simulink model "pulse_heating_official_spine_v04_git_recovery"  (R2025b)
settings: Solver=VariableStepAuto  StartTime=0.0  StopTime=0.001  RelTol=1e-3
PreLoadFcn:
  | addpath('C:\Users\ADMIN\Documents\MATLAB\Examples\R2025b\simscapeelectrical\BatteryThermalManagementExample');
  | addpath('C:\Users\ADMIN\Documents\MATLAB\Examples\R2025b\mcb\SIUnitsExample');
  | addpath('C:\Users\ADMIN\Documents\MATLAB\Examples\R2025b\simscapeelectrical\PMSMDriveThermalExample');
  | load_system('PMSMDriveThermal');
  | set_param('PMSMDriveThermal','SimscapeLogType','none','SimscapeLogSimulationStatistics','off');
  | set_param('PMSMDriveThermal','Dirty','off');
InitFcn:
  | addpath('C:\Users\ADMIN\Documents\MATLAB\Examples\R2025b\simscapeelectrical\BatteryThermalManagementExample');
  | addpath('C:\Users\ADMIN\Documents\MATLAB\Examples\R2025b\mcb\SIUnitsExample');
  | addpath('C:\Users\ADMIN\Documents\MATLAB\Examples\R2025b\simscapeelectrical\PMSMDriveThermalExample');
  | load_system('PMSMDriveThermal');
  | PMSMDriveThermalData;
  | mcb_pmsm_foc_qep_f28379d_SIUnit_data;
  | bw_i = (PI_params.Kp_i + pmsm.Rs) / pmsm.Ld;
  | pmsm.Rs = Rs; pmsm.Ld = Ld; pmsm.Lq = Lq; pmsm.p = N; pmsm.FluxPM = PM;
  | pmsm.J = J; pmsm.Ke = PM*N; pmsm.Kt = 1.5*N*PM;
  | PI_params.Kp_i = bw_i * Ld - Rs; PI_params.Ki_i = bw_i * Rs; PI_params.Ti_i = 1/bw_i;
  | PI_params.Kp_id = PI_params.Kp_i; PI_params.Ki_id = PI_params.Ki_i; PI_params.Ti_id = PI_params.Ti_i;
  | inverter.V_dc = 70; dataType = 'double';
  | BatteryThermalManagementInitialization;
  | ambient=263.15; coolantTemp=263.15; cellT_ini=ambient*ones(1,Ns*Np); cellT_ini4=ambient*ones(1,Ns4*Np4);
model workspace (MAT data in the model file):
  control_status_v4d2_partial_duty_code = 6
  diagnostic_frequency_Hz = 50
  drive_status_v4d2_partial_current_code = 6
  kpi_status_v4d2_partial_numeric_code = 6
  kpi_value_unknown = nan
  limit_factor_unknown_code = 99
  limit_margin_unknown_value = nan
  limit_status_v4c_code = 5
  pulse_command_status_code = 6
  pulse_duty_percent = 50
  pulse_id_amplitude_A = 1
  pulse_iq_amplitude_A = 0
  pulse_mode_code = 4
  pulse_phase_delay_s = 0
undefined symbols (not defined in the file): DiscIntNeverNeededParam, f_losses, Flowrate_vec, fsw, Isc_losses, losses_oc, losses_sc, N, PM, Rs, Ts, Tsc
libraries: fl_lib x36, nesl_utility x33, ee_lib x9, mcbcontrolslib x5, mcbeeMathTransformLib x3, slpidlib x2, simulink x1
(part 1 of 4)
settings Model: Creator=ADMIN  LastModifiedBy=ADMIN
settings DebuggingCC: UnderspecifiedInitializationDetection=Classic
settings SimscapeCC: SimscapeLogType=all  SimscapeLogName=simlog_v4e

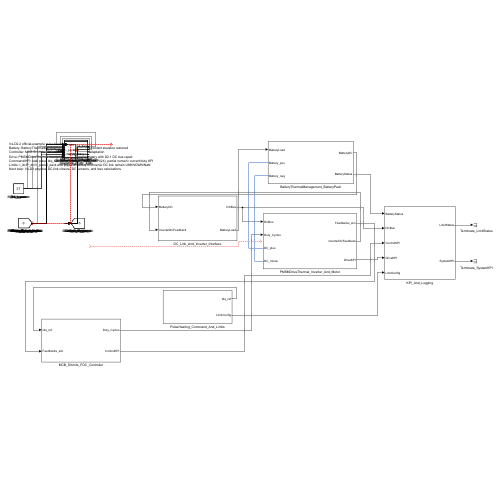
[thumbnail: Simulink's stored preview of the top-level diagram]
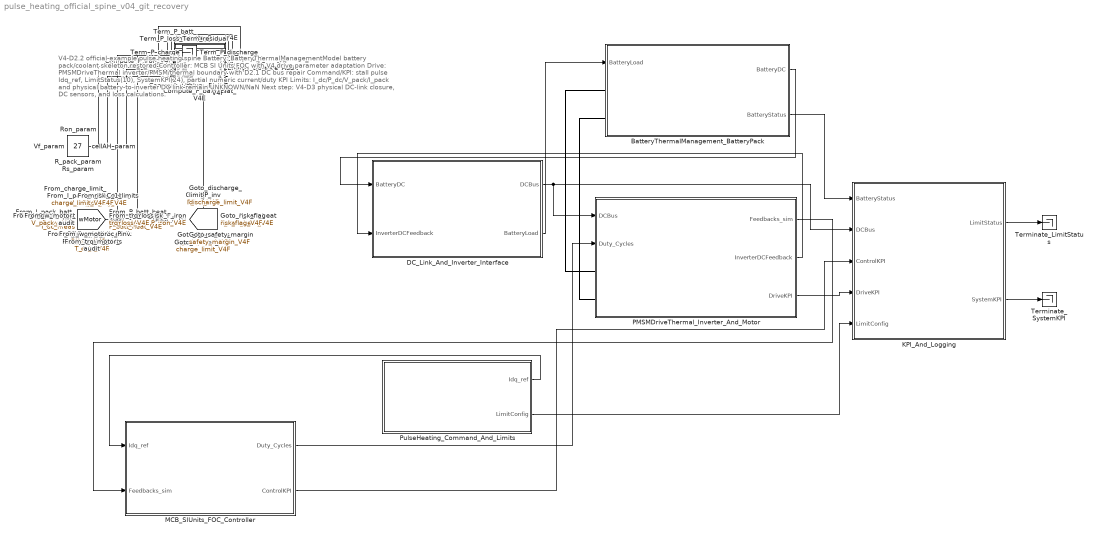
== system pulse_heating_official_spine_v04_git_recovery ==
  note: V4-D2.2 official-example pulse heating spine
      | Battery: BatteryThermalManagementModel battery pack/coolant skeleton restored
      | Controller: MCB SI Units FOC with V4 drive parameter adaptation
      | Drive: PMSMDriveThermal inverter/PMSM/thermal boundary with D2.1 DC bus repair
      | Command/KPI: stall pulse Idq_ref, LimitStatus(10), SystemKPI(24), partial numeric current/duty KPI
      | Limits: I_dc/P_dc/V_pack/I_pack and physical battery-to-inverter DC link remain UNKNOWN/NaN
      | Next step: V4-D3 physical DC-link closure, DC sensors, and loss calculations.
  BatteryThermalManagement_BatteryPack : Subsystem
  Compute_Battery_Limits_V4F : MATLAB Function  TreatAsAtomicUnit=on
  Compute_I_rms_V4G : MATLAB Function  TreatAsAtomicUnit=on
  Compute_Lithium_Risk_V4F : MATLAB Function  TreatAsAtomicUnit=on
  Compute_P_batt_heat_V4E : MATLAB Function  TreatAsAtomicUnit=on
  Compute_P_cu_V4E : MATLAB Function  TreatAsAtomicUnit=on
  Compute_P_inv_V4E : MATLAB Function  TreatAsAtomicUnit=on
  Compute_P_iron_V4E : MATLAB Function  TreatAsAtomicUnit=on
  DC_Link_And_Inverter_Interface : Subsystem
  Energy_Balance_Audit : MATLAB Function  TreatAsAtomicUnit=on
  KPI_And_Logging : Subsystem
  MCB_SIUnits_FOC_Controller : Subsystem
  PMSMDriveThermal_Inverter_And_Motor : Subsystem
  PulseHeating_Command_And_Limits : Subsystem
  R_pack_param : Constant  Value=0.1785
  Ron_param : Constant  Value=0.001
  Rs_param : Constant  Value=Rs
  Term_P_batt_terminal : Terminator
  Term_P_charge : Terminator
  Term_P_discharge : Terminator
  Term_P_loss_total : Terminator
  Term_residual : Terminator
  Terminate_LimitStatus : Terminator
  Terminate_SystemKPI : Terminator
  Vf_param : Constant  Value=0.8
  cellAH_param : Constant  Value=27
  tag scope: I_batt_rms_V4G=global, P_batt_heat_V4E=global, P_cu_V4E=global, P_inv_V4E=global, P_iron_V4E=global, charge_limit_V4F=global, discharge_limit_V4F=global, risk_flag_V4F=global, safety_margin_V4F=global
  wires:
  ? -> ?
  KPI_And_Logging/2(SystemKPI) -> Terminate_SystemKPI/1
  KPI_And_Logging/1(LimitStatus) -> Terminate_LimitStatus/1
  BatteryThermalManagement_BatteryPack/2(BatteryStatus) -> KPI_And_Logging/1(BatteryStatus)
  BatteryThermalManagement_BatteryPack/1(BatteryDC) -> DC_Link_And_Inverter_Interface/1(BatteryDC)
  MCB_SIUnits_FOC_Controller/2(ControlKPI) -> KPI_And_Logging/3(ControlKPI)
  MCB_SIUnits_FOC_Controller/1(Duty_Cycles) -> PMSMDriveThermal_Inverter_And_Motor/2(Duty_Cycles)
  DC_Link_And_Inverter_Interface/2(BatteryLoad) -> BatteryThermalManagement_BatteryPack/1(BatteryLoad)
  DC_Link_And_Inverter_Interface/1(DCBus) -> KPI_And_Logging/2(DCBus), PMSMDriveThermal_Inverter_And_Motor/1(DCBus)
  PMSMDriveThermal_Inverter_And_Motor/3(DriveKPI) -> KPI_And_Logging/4(DriveKPI)
  PMSMDriveThermal_Inverter_And_Motor/2(InverterDCFeedback) -> DC_Link_And_Inverter_Interface/2(InverterDCFeedback)
  PulseHeating_Command_And_Limits/2(LimitConfig) -> KPI_And_Logging/5(LimitConfig)
  PMSMDriveThermal_Inverter_And_Motor/1(Feedbacks_sim) -> MCB_SIUnits_FOC_Controller/2(Feedbacks_sim)
  PulseHeating_Command_And_Limits/1(Idq_ref) -> MCB_SIUnits_FOC_Controller/1(Idq_ref)
  [Idq_debug_V4E] -> Compute_P_cu_V4E/1(Idq_debug)
  Rs_param/1 -> Compute_P_cu_V4E/2(Rs)
  Compute_P_cu_V4E/1(P_cu) -> [P_cu_V4E]
  [trq_loss_V4E] -> Compute_P_iron_V4E/1(trq_loss)
  [wMotor] -> Compute_P_iron_V4E/2(w_motor)
  Compute_P_iron_V4E/1(P_iron) -> [P_iron_V4E]
  [i] -> Compute_P_inv_V4E/1(i_abc)
  Ron_param/1 -> Compute_P_inv_V4E/2(Ron)
  Vf_param/1 -> Compute_P_inv_V4E/3(Vf)
  Compute_P_inv_V4E/1(P_inv) -> [P_inv_V4E]
  [I_dc_meas] -> Compute_P_batt_heat_V4E/1(I_pack)
  R_pack_param/1 -> Compute_P_batt_heat_V4E/2(R_pack)
  Compute_P_batt_heat_V4E/1(P_batt_heat) -> [P_batt_heat_V4E]
  [V_pack_meas] -> Energy_Balance_Audit/1(V_pack)
  [I_dc_meas] -> Energy_Balance_Audit/2(I_pack)
  [P_cu_V4E] -> Energy_Balance_Audit/3(P_cu)
  [P_iron_V4E] -> Energy_Balance_Audit/4(P_iron)
  [P_inv_V4E] -> Energy_Balance_Audit/5(P_inv)
  [P_batt_heat_V4E] -> Energy_Balance_Audit/6(P_batt_heat)
  [wMotor] -> Energy_Balance_Audit/7(w_motor)
  [trqMotor] -> Energy_Balance_Audit/8(trq_motor)
  Energy_Balance_Audit/1(P_batt_terminal) -> Term_P_batt_terminal/1
  Energy_Balance_Audit/2(P_loss_total) -> Term_P_loss_total/1
  Energy_Balance_Audit/3(residual) -> Term_residual/1
  [I_dc_meas] -> Compute_I_rms_V4G/1(I_instant)
  Compute_I_rms_V4G/1(I_rms) -> [I_batt_rms_V4G]
  Energy_Balance_Audit/4(P_charge) -> Term_P_charge/1
  Energy_Balance_Audit/5(P_discharge) -> Term_P_discharge/1
  [T_min_V4F] -> Compute_Battery_Limits_V4F/1(T_min)
  [SOC_1_V4F] -> Compute_Battery_Limits_V4F/2(SOC)
  cellAH_param/1 -> Compute_Battery_Limits_V4F/3(cellAH)
  Compute_Battery_Limits_V4F/1(charge_limit) -> [charge_limit_V4F]
  Compute_Battery_Limits_V4F/2(discharge_limit) -> [discharge_limit_V4F]
  [T_min_V4F] -> Compute_Lithium_Risk_V4F/1(T_min)
  [I_dc_meas] -> Compute_Lithium_Risk_V4F/2(I_pack)
  [charge_limit_V4F] -> Compute_Lithium_Risk_V4F/3(charge_limit)
  Compute_Lithium_Risk_V4F/2(safety_margin) -> [safety_margin_V4F]
  Compute_Lithium_Risk_V4F/1(risk_flag) -> [risk_flag_V4F]
  ? -> ?
  ? -> ?
  ? -> ?
  connections:
  BatteryThermalManagement_BatteryPack/LConn1 -- PMSMDriveThermal_Inverter_And_Motor/LConn1
  BatteryThermalManagement_BatteryPack/LConn2 -- PMSMDriveThermal_Inverter_And_Motor/LConn2

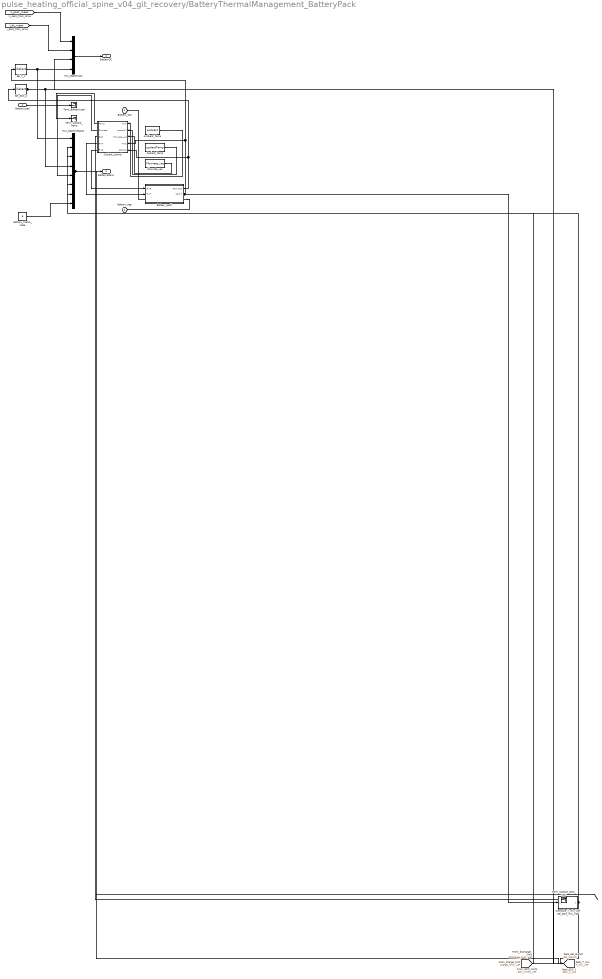
== system pulse_heating_official_spine_v04_git_recovery/BatteryThermalManagement_BatteryPack ==
  BatteryLoad : Inport
  Ambient_Temp : Constant  Value=ambient
  Battery_pack : Subsystem
  Battery_status_code : Constant  Value=4
  Compute_T_min_V4F : MATLAB Function  TreatAsAtomicUnit=on
  Coolant_Temp : Constant  Value=coolantTemp
  Coolant_control : Subsystem
  Flowrate_vec : Constant  Value=Flowrate_vec
  Mux_BatteryDC : Mux
  Mux_BatteryStatus : Mux  Inputs=8
  Sel_SOC_1 : Selector  InputPortWidth=42  IndexOptions=Index vector (dialog)  Indices=1  OutputSizes=1
  Sel_SOC_min_V4F : MATLAB Function  TreatAsAtomicUnit=on
  Sel_T_1 : Selector  InputPortWidth=42  IndexOptions=Index vector (dialog)  Indices=1  OutputSizes=1
  Term_BatteryLoad : Terminator
  Term_Coolant_SOC_new : Terminator
  Term_Coolant_Temp : Terminator
  Battery_pos : PMIOPort  Side=Left
  Battery_neg : PMIOPort  Port=2  Side=Left
  BatteryDC : Outport
  BatteryStatus : Outport  Port=2
  tag scope: SOC_1_V4F=global, T_min_V4F=global, bat_branch=global
  wires:
  Battery_pack/1(Pack SOC) -> Sel_SOC_1/1, Coolant_control/5(SOCvec)
  [V_pack_meas] -> Mux_BatteryDC/1
  Sel_T_1/1 -> Mux_BatteryDC/4, Mux_BatteryStatus/1
  [I_dc_meas] -> Mux_BatteryDC/2
  Sel_SOC_1/1 -> Mux_BatteryDC/3, Mux_BatteryStatus/4, [SOC_1_V4F]
  BatteryLoad/1 -> Term_BatteryLoad/1
  Battery_status_code/1 -> Mux_BatteryStatus/8
  Mux_BatteryDC/1 -> BatteryDC/1
  Mux_BatteryStatus/1 -> BatteryStatus/1, [bat_branch]
  Coolant_control/5(FlwR) -> Battery_pack/1(FlwR)
  Coolant_control/4(FlwT) -> Battery_pack/2(FlwT)
  Coolant_control/2(Flowrate) -> Mux_BatteryStatus/5
  Coolant_control/1(Temp) -> Term_Coolant_Temp/1
  Ambient_Temp/1 -> Coolant_control/1(Amb)
  Coolant_Temp/1 -> Coolant_control/2(coolant T)
  Flowrate_vec/1 -> Coolant_control/3(Flowrate_vec)
  Battery_pack/2(Pack T) -> Sel_T_1/1, Coolant_control/4(Tvec), Compute_T_min_V4F/1(Pack_T)
  Compute_T_min_V4F/1(T_min) -> Mux_BatteryStatus/2, [T_min_V4F]
  [charge_limit_V4F] -> Mux_BatteryStatus/6
  [discharge_limit_V4F] -> Mux_BatteryStatus/7
  [SOC_limits_V4F] -> Sel_SOC_min_V4F/1(SOC_limits)
  Sel_SOC_min_V4F/1(SOC_min) -> Mux_BatteryStatus/3
  Coolant_control/3(SOC) -> Term_Coolant_SOC_new/1
  connections:
  Battery_pack/RConn1 -- Battery_neg/RConn1
  Battery_pack/LConn1 -- Battery_pos/RConn1

== system pulse_heating_official_spine_v04_git_recovery/DC_Link_And_Inverter_Interface ==
  BatteryDC : Inport
  InverterDCFeedback : Inport  Port=2
  Sel_Battery_V_pack : Selector  InputPortWidth=4  IndexOptions=Index vector (dialog)  Indices=1  OutputSizes=1
  Sel_Inverter_I_dc : Selector  InputPortWidth=4  IndexOptions=Index vector (dialog)  Indices=2  OutputSizes=1
  DCBus : Outport
  BatteryLoad : Outport  Port=2
  wires:
  Sel_Inverter_I_dc/1 -> BatteryLoad/1
  BatteryDC/1 -> Sel_Battery_V_pack/1
  InverterDCFeedback/1 -> Sel_Inverter_I_dc/1
  Sel_Battery_V_pack/1 -> DCBus/1

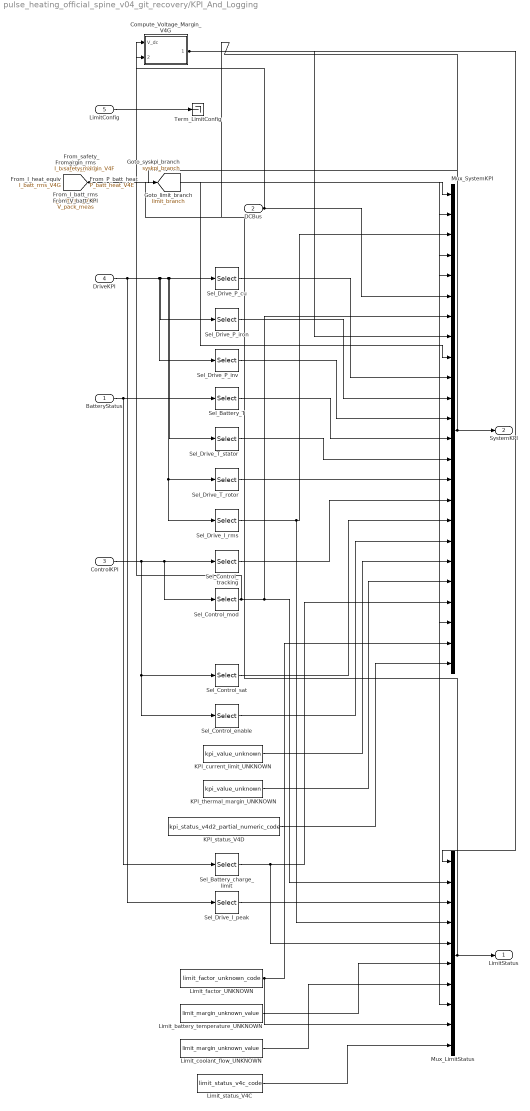
== system pulse_heating_official_spine_v04_git_recovery/KPI_And_Logging ==
  BatteryStatus : Inport
  DCBus : Inport  Port=2
  ControlKPI : Inport  Port=3
  DriveKPI : Inport  Port=4
  LimitConfig : Inport  Port=5
  Compute_Voltage_Margin_V4G : MATLAB Function  TreatAsAtomicUnit=on
  KPI_current_limit_UNKNOWN : Constant  Value=kpi_value_unknown
  KPI_status_V4D : Constant  Value=kpi_status_v4d2_partial_numeric_code
  KPI_thermal_margin_UNKNOWN : Constant  Value=kpi_value_unknown
  Limit_battery_temperature_UNKNOWN : Constant  Value=limit_margin_unknown_value
  Limit_coolant_flow_UNKNOWN : Constant  Value=limit_margin_unknown_value
  Limit_factor_UNKNOWN : Constant  Value=limit_factor_unknown_code
  Limit_status_V4C : Constant  Value=limit_status_v4c_code
  Mux_LimitStatus : Mux  Inputs=10
  Mux_SystemKPI : Mux  Inputs=24
  Sel_Battery_T : Selector  InputPortWidth=8  IndexOptions=Index vector (dialog)  Indices=1  OutputSizes=1
  Sel_Battery_charge_limit : Selector  InputPortWidth=8  IndexOptions=Index vector (dialog)  Indices=6  OutputSizes=1
  Sel_Control_enable : Selector  InputPortWidth=5  IndexOptions=Index vector (dialog)  Indices=4  OutputSizes=1
  Sel_Control_mod : Selector  InputPortWidth=5  IndexOptions=Index vector (dialog)  Indices=2  OutputSizes=1
  Sel_Control_sat : Selector  InputPortWidth=5  IndexOptions=Index vector (dialog)  Indices=3  OutputSizes=1
  Sel_Control_tracking : Selector  InputPortWidth=5  IndexOptions=Index vector (dialog)  Indices=1  OutputSizes=1
  Sel_Drive_I_peak : Selector  InputPortWidth=8  IndexOptions=Index vector (dialog)  Indices=2  OutputSizes=1
  Sel_Drive_I_rms : Selector  InputPortWidth=8  IndexOptions=Index vector (dialog)  Indices=1  OutputSizes=1
  Sel_Drive_P_cu : Selector  InputPortWidth=8  IndexOptions=Index vector (dialog)  Indices=3  OutputSizes=1
  Sel_Drive_P_inv : Selector  InputPortWidth=8  IndexOptions=Index vector (dialog)  Indices=5  OutputSizes=1
  Sel_Drive_P_iron : Selector  InputPortWidth=8  IndexOptions=Index vector (dialog)  Indices=4  OutputSizes=1
  Sel_Drive_T_rotor : Selector  InputPortWidth=8  IndexOptions=Index vector (dialog)  Indices=7  OutputSizes=1
  Sel_Drive_T_stator : Selector  InputPortWidth=8  IndexOptions=Index vector (dialog)  Indices=6  OutputSizes=1
  Term_LimitConfig : Terminator
  LimitStatus : Outport
  SystemKPI : Outport  Port=2
  tag scope: limit_branch=global, syskpi_branch=global
  wires:
  KPI_current_limit_UNKNOWN/1 -> Mux_SystemKPI/19
  Sel_Drive_T_stator/1 -> Mux_SystemKPI/14
  ControlKPI/1 -> Sel_Control_enable/1, Sel_Control_sat/1, Sel_Control_tracking/1, Sel_Control_mod/1
  Limit_status_V4C/1 -> Mux_LimitStatus/10
  KPI_thermal_margin_UNKNOWN/1 -> Mux_SystemKPI/20
  BatteryStatus/1 -> Sel_Battery_T/1, Sel_Battery_charge_limit/1
  Sel_Drive_I_rms/1 -> Mux_LimitStatus/4, Mux_SystemKPI/3
  LimitConfig/1 -> Term_LimitConfig/1
  DCBus/1 -> Mux_SystemKPI/6, Compute_Voltage_Margin_V4G/1(V_dc)
  Mux_SystemKPI/1 -> SystemKPI/1, [syskpi_branch]
  DriveKPI/1 -> Sel_Drive_T_rotor/1, Sel_Drive_I_rms/1, Sel_Drive_P_cu/1, Sel_Drive_T_stator/1, Sel_Drive_P_iron/1, Sel_Drive_P_inv/1, Sel_Drive_I_peak/1
  Sel_Battery_T/1 -> Mux_SystemKPI/13
  Sel_Drive_P_cu/1 -> Mux_SystemKPI/10
  Sel_Control_enable/1 -> Mux_SystemKPI/18
  Sel_Drive_P_iron/1 -> Mux_SystemKPI/11
  Sel_Drive_P_inv/1 -> Mux_SystemKPI/12
  Sel_Drive_T_rotor/1 -> Mux_SystemKPI/15
  Limit_battery_temperature_UNKNOWN/1 -> Mux_LimitStatus/6
  Sel_Control_tracking/1 -> Mux_SystemKPI/16
  Sel_Control_mod/1 -> Mux_LimitStatus/2, Mux_SystemKPI/7, Compute_Voltage_Margin_V4G/2(mod_index)
  Sel_Control_sat/1 -> Mux_SystemKPI/17
  KPI_status_V4D/1 -> Mux_SystemKPI/24
  Sel_Battery_charge_limit/1 -> Mux_LimitStatus/5, Mux_SystemKPI/21
  Sel_Drive_I_peak/1 -> Mux_LimitStatus/3
  Limit_factor_UNKNOWN/1 -> Mux_LimitStatus/9, Mux_SystemKPI/23
  Limit_coolant_flow_UNKNOWN/1 -> Mux_LimitStatus/7
  Mux_LimitStatus/1 -> LimitStatus/1, [limit_branch]
  [P_batt_heat_V4E] -> Mux_SystemKPI/9
  [V_pack_meas] -> Mux_SystemKPI/5
  [I_batt_rms_V4G] -> Mux_SystemKPI/1
  [I_batt_rms_V4G] -> Mux_SystemKPI/2
  [I_batt_rms_V4G] -> Mux_SystemKPI/4
  Compute_Voltage_Margin_V4G/1(V_margin) -> Mux_LimitStatus/1, Mux_SystemKPI/8
  [safety_margin_V4F] -> Mux_LimitStatus/8, Mux_SystemKPI/22

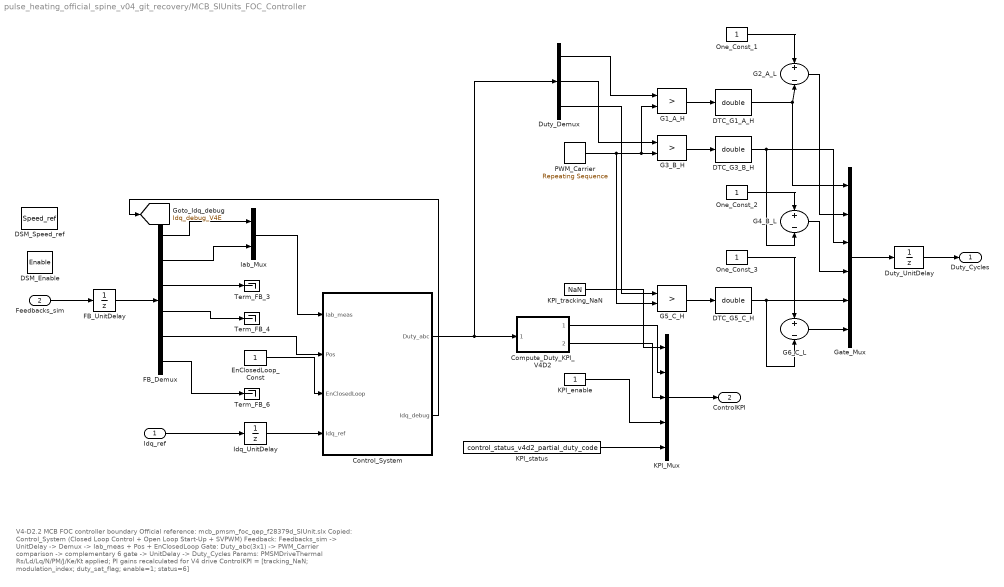
== system pulse_heating_official_spine_v04_git_recovery/MCB_SIUnits_FOC_Controller ==
  note: V4-D2.2 MCB FOC controller boundary
      | Official reference: mcb_pmsm_foc_qep_f28379d_SIUnit.slx
      | Copied: Control_System (Closed Loop Control + Open Loop Start-Up + SVPWM)
      | Feedback: Feedbacks_sim -> UnitDelay -> Demux -> Iab_meas + Pos + EnClosedLoop
      | Gate: Duty_abc(3x1) -> PWM_Carrier comparison -> complementary 6 gate -> UnitDelay -> Duty_Cycles
      | Params: PMSMDriveThermal Rs/Ld/Lq/N/PM/J/Ke/Kt applied; PI gains recalculated for V4 drive
      | ControlKPI = [tracking_NaN; modulation_index; duty_sat_flag; enable=1; status=6]
  Idq_ref : Inport
  Feedbacks_sim : Inport  Port=2
  Compute_Duty_KPI_V4D2 : MATLAB Function  TreatAsAtomicUnit=on
  Control_System : Subsystem  TreatAsAtomicUnit=on
  DSM_Enable : DataStoreMemory  DataStoreName=Enable  WriteAfterWriteMsg=warning  InitialValue=1  ShowAdditionalParam=off
  DSM_Speed_ref : DataStoreMemory  DataStoreName=Speed_ref  WriteAfterWriteMsg=warning  ShowAdditionalParam=off
  DTC_G1_A_H : DataTypeConversion  OutDataTypeStr=double  SaturateOnIntegerOverflow=off  RndMeth=Floor
  DTC_G3_B_H : DataTypeConversion  OutDataTypeStr=double  SaturateOnIntegerOverflow=off  RndMeth=Floor
  DTC_G5_C_H : DataTypeConversion  OutDataTypeStr=double  SaturateOnIntegerOverflow=off  RndMeth=Floor
  Duty_Demux : Demux  Outputs=3
  Duty_UnitDelay : UnitDelay  SampleTime=Tsc  HasFrameUpgradeWarning=on
  EnClosedLoop_Const : Constant
  FB_Demux : Demux  Outputs=6
  FB_UnitDelay : UnitDelay  SampleTime=Tsc  HasFrameUpgradeWarning=on
  G1_A_H : RelationalOperator  Operator=>  OutDataTypeStr=boolean  RndMeth=Simplest  InputSameDT=off
  G2_A_L : Sum  Inputs=+-
  G3_B_H : RelationalOperator  Operator=>  OutDataTypeStr=boolean  RndMeth=Simplest  InputSameDT=off
  G4_B_L : Sum  Inputs=+-
  G5_C_H : RelationalOperator  Operator=>  OutDataTypeStr=boolean  RndMeth=Simplest  InputSameDT=off
  G6_C_L : Sum  Inputs=+-
  Gate_Mux : Mux  Inputs=6
  Iab_Mux : Mux  Inputs=2
  Idq_UnitDelay : UnitDelay  SampleTime=Tsc  HasFrameUpgradeWarning=on
  KPI_Mux : Mux  Inputs=5
  KPI_enable : Constant
  KPI_status : Constant  Value=control_status_v4d2_partial_duty_code
  KPI_tracking_NaN : Constant  Value=NaN
  One_Const_1 : Constant
  One_Const_2 : Constant
  One_Const_3 : Constant
  PWM_Carrier : simulink/Sources/Repeating Sequence  rep_seq_t=[0 1/fsw]  rep_seq_y=[0 1]
  Term_FB_3 : Terminator
  Term_FB_4 : Terminator
  Term_FB_6 : Terminator
  Duty_Cycles : Outport
  ControlKPI : Outport  Port=2
  tag scope: Idq_debug_V4E=global
  wires:
  Feedbacks_sim/1 -> FB_UnitDelay/1
  FB_Demux/5 -> Control_System/2(Pos)
  G2_A_L/1 -> Gate_Mux/2
  DTC_G3_B_H/1 -> G4_B_L/2, Gate_Mux/3
  FB_Demux/1 -> Iab_Mux/1
  G4_B_L/1 -> Gate_Mux/4
  Duty_Demux/3 -> G5_C_H/1
  FB_UnitDelay/1 -> FB_Demux/1
  KPI_Mux/1 -> ControlKPI/1
  FB_Demux/6 -> Term_FB_6/1
  FB_Demux/2 -> Iab_Mux/2
  FB_Demux/3 -> Term_FB_3/1
  Control_System/1(Duty_abc) -> Duty_Demux/1, Compute_Duty_KPI_V4D2/1(duty_abc)
  FB_Demux/4 -> Term_FB_4/1
  Idq_ref/1 -> Idq_UnitDelay/1
  One_Const_1/1 -> G2_A_L/1
  Iab_Mux/1 -> Control_System/1(Iab_meas)
  DTC_G1_A_H/1 -> G2_A_L/2, Gate_Mux/1
  EnClosedLoop_Const/1 -> Control_System/3(EnClosedLoop)
  Idq_UnitDelay/1 -> Control_System/4(Idq_ref)
  Duty_Demux/1 -> G1_A_H/1
  Duty_Demux/2 -> G3_B_H/1
  KPI_tracking_NaN/1 -> KPI_Mux/1
  PWM_Carrier/1 -> G1_A_H/2, G3_B_H/2, G5_C_H/2
  Compute_Duty_KPI_V4D2/1(mod_index) -> KPI_Mux/2
  Compute_Duty_KPI_V4D2/2(sat_flag) -> KPI_Mux/3
  KPI_enable/1 -> KPI_Mux/4
  One_Const_3/1 -> G6_C_L/1
  KPI_status/1 -> KPI_Mux/5
  G5_C_H/1 -> DTC_G5_C_H/1
  G1_A_H/1 -> DTC_G1_A_H/1
  G3_B_H/1 -> DTC_G3_B_H/1
  G6_C_L/1 -> Gate_Mux/6
  One_Const_2/1 -> G4_B_L/1
  DTC_G5_C_H/1 -> G6_C_L/2, Gate_Mux/5
  Gate_Mux/1 -> Duty_UnitDelay/1
  Duty_UnitDelay/1 -> Duty_Cycles/1
  Control_System/2(Idq_debug) -> [Idq_debug_V4E]

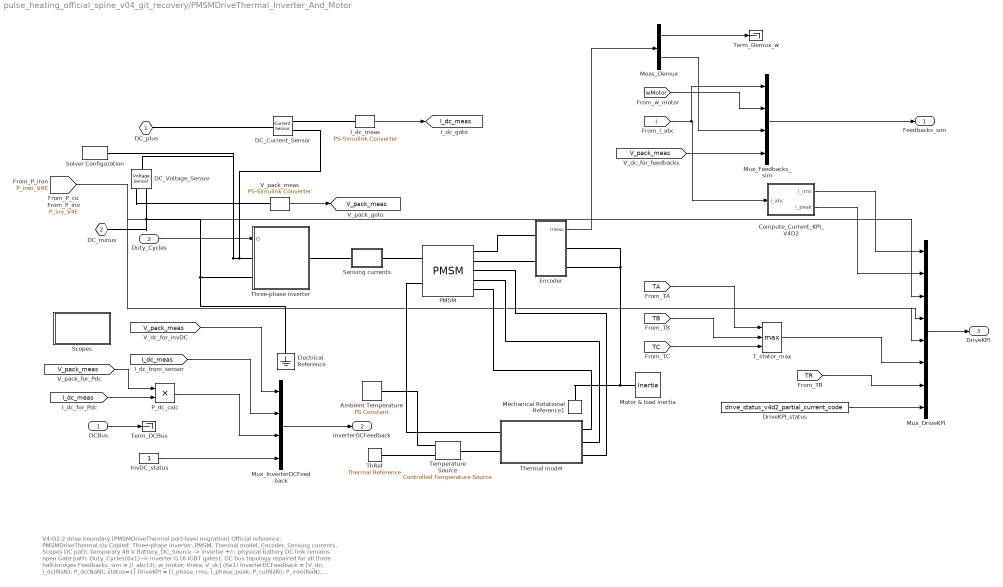
== system pulse_heating_official_spine_v04_git_recovery/PMSMDriveThermal_Inverter_And_Motor ==
  note: V4-D2.2 drive boundary (PMSMDriveThermal port-level migration)
      | Official reference: PMSMDriveThermal.slx
      | Copied: Three-phase inverter, PMSM, Thermal model, Encoder, Sensing currents, Scopes
      | DC path: temporary 48 V Battery_DC_Source -> inverter +/-; physical battery DC link remains open
      | Gate path: Duty_Cycles(6x1) -> inverter G (6 IGBT gates); DC bus topology repaired for all three half-bridges
      | Feedbacks_sim = [i_abc(3); w_motor; theta; V_dc] (6x1)
      | InverterDCFeedback = [V_dc; I_dc(NaN); P_dc(NaN); status=1]
      | DriveKPI = [I_phase_rms; I_phase_peak; P_cu(NaN); P_iron(NaN); P_inv(NaN); T_stator; T_rotor; status=6]
  DCBus : Inport
  Duty_Cycles : Inport  Port=2
  Ambient Temperature : fl_lib/Physical Signals/Sources/PS Constant  constant=300.15 K
  Compute_Current_KPI_V4D2 : MATLAB Function  TreatAsAtomicUnit=on
  DC_Current_Sensor : fl_lib/Electrical/Electrical Sensors/Current Sensor
  DC_Voltage_Sensor : fl_lib/Electrical/Electrical Sensors/Voltage Sensor
  DriveKPI_status : Constant  Value=drive_status_v4d2_partial_current_code
  Electrical Reference : fl_lib/Electrical/Electrical Elements/Electrical Reference
  Encoder : Subsystem
  I_dc_meas : nesl_utility/PS-Simulink Converter  PhysicalDomain=network_engine_domain  SubClassName=ps_output  LeftPortType=input  RightPortType=output  PseudoPeriodic=off  Frequencies=[]  VectorFormat=inherit  Unit=inherit  AffineConversion=off
  InvDC_status : Constant
  Meas_Demux : Demux  Outputs=2
  Mechanical Rotational Reference1 : fl_lib/Mechanical/Rotational Elements/Mechanical Rotational Reference
  Motor & load inertia : fl_lib/Mechanical/Rotational Elements/Inertia  inertia=J kg*m^2  num_ports=foundation.enum.numPorts2.one  w_specify=on  w_priority=High  w=0 rpm  w_nominal_specify=off  w_nominal_value=1  w_nominal_unit=rad/s  t_specify=off  t_priority=High  t=0 N*m  t_nominal_specify=off  t_nominal_value=1  t_nominal_unit=N*m
  Mux_DriveKPI : Mux  Inputs=8
  Mux_Feedbacks_sim : Mux
  Mux_InverterDCFeedback : Mux
  PMSM : ee_lib/Electromechanical/Permanent Magnet/PMSM  port_option=ee.enum.threePhasePort.composite  winding_type=ee.enum.statorconnection.wye  machine_param=ee.enum.pmsm.parameterization.constant  nPolePairs=N  pmflux_param=ee.enum.pmflux.fluxlinkage  pm_flux_linkage=PM Wb  torque_constant=0.18 N*m/A  back_emf_constant=0.18 V/(rad/s)  stator_param=ee.enum.statorparam.LdLqL0  Ld=Ld H  Lq=Lq H  idVec=[-200, 0, 200] A  iqVec=[-200, 0, 200] A  LdMatrix=0.0002 * ones(3, 3) H  LqMatrix=0.0002 * ones(3, 3) H  PmMatrix=0.1 * ones(3, 3) Wb  ktMatrix=0.18 * ones(3, 3) N*m/A  keMatrix=0.18 * ones(3, 3) V/(rad/s)  L0=L0 H  Ls=0.0002 H  Lm=0.00002 H  Ms=0.00002 H  Rs=Rs Ohm  zero_sequence=ee.enum.park.zerosequence.exclude  axes_param=ee.enum.rotorangle.qaxis  loss_param=ee.enum.ironloss.empirical  losses_oc=losses_oc W  losses_sc=losses_sc W  f_losses=f_losses Hz  Isc_losses=Isc_losses A  J=0 kg*m^2  lam=0 N*m/(rad/s)  i_d_specify=off  i_d_priority=None  i_d=0 A  i_d_nominal_specify=off  i_d_nominal_value=1  i_d_nominal_unit=A  i_q_specify=off  i_q_priority=None  i_q=0 A  i_q_nominal_specify=off  i_q_nominal_value=1  i_q_nominal_unit=A  torque_specify=off  torque_priority=None  torque=0 N*m  torque_nominal_specify=off  torque_nominal_value=1  torque_nominal_unit=N*m  angular_velocity_specify=on  angular_velocity_priority=None  angular_velocity=0 rpm  angular_velocity_nominal_specify=off  angular_velocity_nominal_value=1  angular_velocity_nominal_unit=rpm  angular_position_specify=on  angular_position_priority=High  angular_position=0 rad  angular_position_nominal_specify=off  angular_position_nominal_value=1  angular_position_nominal_unit=deg  alpha=alpha 1/K  alpha_flux=alpha_flux 1/K  Tmeas=Tmeas K  stator_thermal_mass=stator_thermal_mass J/K  rotor_thermal_mass=rotor_thermal_mass J/K  Rm_percent_rotor=Rm_percent_rotor  Rd_percent_rotor=Rd_percent_rotor  temperatureA_specify=off  temperatureA_priority=High  temperatureA=25 degC  temperatureA_nominal_specify=off  temperatureA_nominal_value=1  temperatureA_nominal_unit=degC  temperatureB_specify=off  temperatureB_priority=High  temperatureB=25 degC  temperatureB_nominal_specify=off  temperatureB_nominal_value=1  temperatureB_nominal_unit=degC  temperatureC_specify=off  temperatureC_priority=High  temperatureC=25 degC  temperatureC_nominal_specify=off  temperatureC_nominal_value=1  temperatureC_nominal_unit=degC  temperatureR_specify=off  temperatureR_priority=High  temperatureR=25 degC  temperatureR_nominal_specify=off  temperatureR_nominal_value=1  temperatureR_nominal_unit=degC
      settings: InternalSimscapePortConfiguration="{\"Bottom\":[],\"Left\":[{\"id\":\"N\",\"label\":\"~\",\"type\":\"foundation.electrical.three_phase\"},{\"id\":\"HR\",\"label\":\"HR\",\"type\":\"foundation.thermal.thermal\"}],\"Right\":[{\"id\":\"R\",\"label\":\"R\",\"type\":\"foundation.mechanical.rotational.rotational\"},{\"id\":\"C\",\"label\":\"C\",\"type\":\"foundation.mechanical.rotational.rotational\"},{\"id\":\"HA\",\"label\":\"HA\",\"type\":\"foundation.thermal.thermal\"},{\"id\":\"HB\",\"label\":\"HB\",\"type\":\"foundation.thermal.thermal\"},{\"id\":\"HC\",\"label\":\"HC\",\"type\":\"foundation.thermal.thermal\"}],\"Top\":[]}"
  P_dc_calc : Product
  Scopes : Subsystem
  Sensing currents : Subsystem
      mask Display: disp('i')
  Solver Configuration : nesl_utility/Solver Configuration  PhysicalDomain=network_engine_domain  SubClassName=solver  LeftPortType=input  RightPortType=generic  Tones=[]  Harmonics=[]  SimulateNoise=off  Profile=off  UseLocalSampling=off  EnableSwitchedLinearOptims=on  FrequencyDomain=off  UseCCode=off  RelTol=0.001  AbsTol=1e-06  MinStep=1e-09  ToWorkspace=off  RevertToSquareIcSolve=off  NumHomotopyIterations=100  PhasorMode=off  PhasorModeNumHarmonics=1  ConsistencySolver=NEWTON_FTOL  IndexReductionMethod=DerivativeReplacement  DoDC=off  ResidualTolerance=1e-9  ConsistencyTolSource=GLOBAL  ConsistencyAbsTol=0.001  ConsistencyRelTol=0.001  ConsistencyTolFactor=0.001  UseLocalSolver=on  LocalSolverChoice=NE_BACKWARD_EULER_ADVANCER  ResolveIndetEquations=on  FunctionEvalNumThread=1  LocalSolverSampleTime=Ts  DoFixedCost=on  MaxNonlinIter=6  MaxModeIter=2  ComputeImpulses=off  ImpulseIterations=2  LinearAlgebra=auto  LinearAlgebraNumThread=0  EquationFormulation=NE_TIME_EF  DelaysMemoryBudget=1024  AutomaticFiltering=on  FilteringTimeConstant=0.001  PartitionStorageMethod=AS_NEEDED  PartitionMemoryBudget=1024  PartitionMethod=FAST  MultibodyUseLocalSolver=off  MultibodyLocalSolverChoice=ODE1  MultibodyLocalSolverSampleTime=0.001
  T_stator_max : MinMax  Function=max  Inputs=3
  Temperature Source : fl_lib/Thermal/Thermal Sources/Controlled Temperature Source
  Term_DCBus : Terminator
  Term_Demux_w : Terminator
  ThRef : fl_lib/Thermal/Thermal Elements/Thermal Reference
  Thermal model : Subsystem  Tag=PublishSubsystem
  Three-phase inverter : Subsystem
  V_pack_meas : nesl_utility/PS-Simulink Converter  PhysicalDomain=network_engine_domain  SubClassName=ps_output  LeftPortType=input  RightPortType=output  PseudoPeriodic=off  Frequencies=[]  VectorFormat=inherit  Unit=inherit  AffineConversion=off
  DC_plus : PMIOPort  Side=Left
  DC_minus : PMIOPort  Port=2  Side=Left
  Feedbacks_sim : Outport
  InverterDCFeedback : Outport  Port=2
  DriveKPI : Outport  Port=3
  tag scope: I_dc_meas=global, V_pack_meas=global
  wires:
  Compute_Current_KPI_V4D2/2(i_peak) -> Mux_DriveKPI/2
  Meas_Demux/1 -> Term_Demux_w/1
  V_pack_meas/1 -> [V_pack_meas]
  DCBus/1 -> Term_DCBus/1
  [V_pack_meas] -> Mux_Feedbacks_sim/4
  [I_dc_meas] -> P_dc_calc/2
  [V_pack_meas] -> P_dc_calc/1
  Mux_DriveKPI/1 -> DriveKPI/1
  Compute_Current_KPI_V4D2/1(i_rms) -> Mux_DriveKPI/1
  InvDC_status/1 -> Mux_InverterDCFeedback/4
  Duty_Cycles/1 -> Three-phase inverter/1(G)
  [V_pack_meas] -> Mux_InverterDCFeedback/1
  I_dc_meas/1 -> [I_dc_meas]
  [I_dc_meas] -> Mux_InverterDCFeedback/2
  P_dc_calc/1 -> Mux_InverterDCFeedback/3
  Mux_InverterDCFeedback/1 -> InverterDCFeedback/1
  [i] -> Mux_Feedbacks_sim/1, Compute_Current_KPI_V4D2/1(i_abc)
  Encoder/1(meas) -> Meas_Demux/1
  DriveKPI_status/1 -> Mux_DriveKPI/8
  Meas_Demux/2 -> Mux_Feedbacks_sim/3
  [wMotor] -> Mux_Feedbacks_sim/2
  [TA] -> T_stator_max/1
  [TB] -> T_stator_max/2
  [TC] -> T_stator_max/3
  Mux_Feedbacks_sim/1 -> Feedbacks_sim/1
  T_stator_max/1 -> Mux_DriveKPI/6
  [TR] -> Mux_DriveKPI/7
  [P_cu_V4E] -> Mux_DriveKPI/3
  [P_iron_V4E] -> Mux_DriveKPI/4
  [P_inv_V4E] -> Mux_DriveKPI/5
  connections:
  DC_Voltage_Sensor/RConn1 -- V_pack_meas/LConn1
  DC_plus/RConn1 -- DC_Current_Sensor/LConn1
  DC_Voltage_Sensor/RConn2 -- Electrical Reference/LConn1 -- Three-phase inverter/LConn2 -- DC_minus/RConn1
  DC_Voltage_Sensor/LConn1 -- Three-phase inverter/LConn1 -- DC_Current_Sensor/RConn2 -- Solver Configuration/RConn1
  Sensing currents/RConn1 -- PMSM/LConn1
  DC_Current_Sensor/RConn1 -- I_dc_meas/LConn1
  Three-phase inverter/RConn1 -- Sensing currents/LConn1
  ThRef/LConn1 -- Temperature Source/RConn2
  Ambient Temperature/RConn1 -- Temperature Source/RConn1
  PMSM/LConn2 -- Thermal model/LConn1
  PMSM/RConn1 -- Encoder/LConn1
  PMSM/RConn2 -- Encoder/LConn2
  PMSM/RConn3 -- Thermal model/RConn3
  PMSM/RConn4 -- Thermal model/RConn2
  PMSM/RConn5 -- Thermal model/RConn1
  Temperature Source/LConn1 -- Thermal model/LConn2
  Motor & load inertia/LConn1 -- Encoder/RConn1 -- Encoder/RConn2 -- Mechanical Rotational Reference1/LConn1

== system pulse_heating_official_spine_v04_git_recovery/PulseHeating_Command_And_Limits ==
  Id_Pulse_Stall : DiscretePulseGenerator  PulseType=Time based  Period=1/diagnostic_frequency_Hz  PulseWidth=pulse_duty_percent  PhaseDelay=pulse_phase_delay_s
  Iq_ref_zero_A : Constant  Value=pulse_iq_amplitude_A
  Limit_Duty_Percent : Constant  Value=pulse_duty_percent
  Limit_Frequency_Hz : Constant  Value=diagnostic_frequency_Hz
  Limit_Id_A : Constant  Value=pulse_id_amplitude_A
  Limit_Mode_Code : Constant  Value=pulse_mode_code
  Limit_Phase_Delay_s : Constant  Value=pulse_phase_delay_s
  Limit_Status_Code : Constant  Value=pulse_command_status_code
  Mux_Idq_ref : Mux  Inputs=2
  Mux_LimitConfig : Mux  Inputs=6
  Offset_To_Negative_A : Bias  Bias=-pulse_id_amplitude_A  SaturateOnIntegerOverflow=off
  Scale_To_Bipolar_A : Gain  Gain=2*pulse_id_amplitude_A
  Idq_ref : Outport
  LimitConfig : Outport  Port=2
  wires:
  Limit_Duty_Percent/1 -> Mux_LimitConfig/3
  Limit_Id_A/1 -> Mux_LimitConfig/1
  Iq_ref_zero_A/1 -> Mux_Idq_ref/2
  Limit_Mode_Code/1 -> Mux_LimitConfig/5
  Limit_Frequency_Hz/1 -> Mux_LimitConfig/2
  Mux_LimitConfig/1 -> LimitConfig/1
  Id_Pulse_Stall/1 -> Scale_To_Bipolar_A/1
  Limit_Phase_Delay_s/1 -> Mux_LimitConfig/4
  Limit_Status_Code/1 -> Mux_LimitConfig/6
  Scale_To_Bipolar_A/1 -> Offset_To_Negative_A/1
  Offset_To_Negative_A/1 -> Mux_Idq_ref/1
  Mux_Idq_ref/1 -> Idq_ref/1
